simulink model "jawkj"  (R2015a)
settings: Solver=ode45  StartTime=0.0  StopTime=10.0  RelTol=1e-3
libraries: fl_lib x6
settings Model: Creator=AMDIS  LastModifiedBy=AMDIS

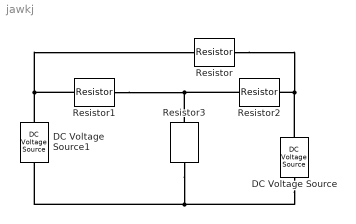
== system jawkj ==
  DC Voltage Source : fl_lib/Electrical/Electrical Sources/DC Voltage Source  v0=1 V
  DC Voltage Source1 : fl_lib/Electrical/Electrical Sources/DC Voltage Source  v0=1 V
  Resistor{,1..3} (4 alike) : fl_lib/Electrical/Electrical Elements/Resistor  R=1 Ohm  i_specify=off  i_priority=High  i=0 A  v_specify=off  v_priority=High  v=0 V
  connections:
  Resistor1/LConn1 -- DC Voltage Source1/LConn1 -- Resistor/LConn1
  Resistor1/RConn1 -- Resistor3/LConn1 -- Resistor2/LConn1
  Resistor/RConn1 -- DC Voltage Source/LConn1 -- Resistor2/RConn1
  Resistor3/RConn1 -- DC Voltage Source1/RConn1 -- DC Voltage Source/RConn1
